simulink model "Environmentmodel"  (R2024a)
settings: Solver=VariableStepAuto  StartTime=0.0  StopTime=10.0  RelTol=1e-3
undefined symbols (not defined in the file or in its folder): F, Light, MIL, quad
libraries: shared6dof x1, aerolibwind2 x1
settings Model: Creator=akulramasubban  LastModifiedBy=akulramasubban

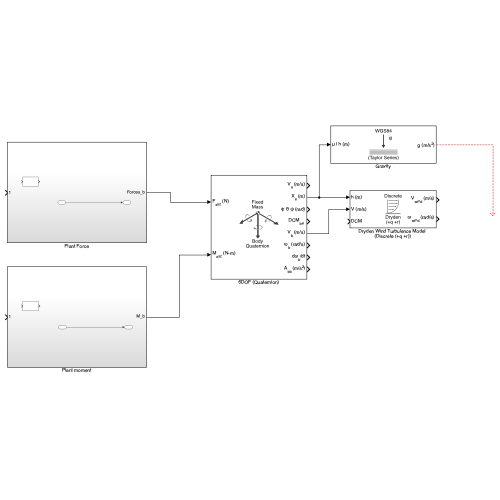
[thumbnail: Simulink's stored preview of the top-level diagram]
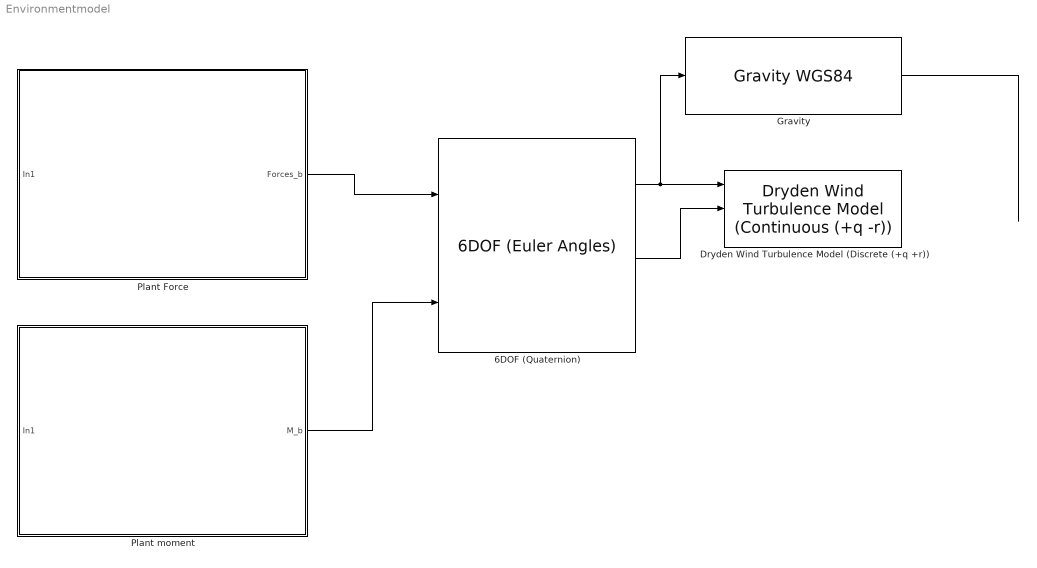
== system Environmentmodel ==
  6DOF (Quaternion) : shared6dof/6DOF (Euler Angles)  units=Metric (MKS)  mtype=Fixed  rep=Quaternion  xme_0=IC.pos  Vm_0=IC.vel  eul_0=IC.euler  pm_0=IC.omegaB  mass_0=quad  mass_e=0.5  mass_f=2.0  inertia=[quad(1,1), quad(2,2), quad(3,3)]  inertia_e=eye(3)  inertia_f=2*eye(3)  k_quat=1.0  vre_flag=on  abi_flag=off  aMode=0  xme_statename=''  Vm_statename=''  eul_statename=''  quat_statename=''  pm_statename=''  mass_statename=''
      settings: LibrarySourceBlock=aerolib6dof2/6DOF (Quaternion)
  Dryden Wind Turbulence Model (Discrete (+q +r)) : aerolibwind2/Dryden Wind Turbulence Model  (Continuous (+q -r))  units=Metric (MKS)  spec=MIL-F-8785C  model=Discrete Dryden (+q +r)  W20=15  Wdeg=0  TurbProb=10^-2 - Light  L_high=533.4  Wingspan=10  ts=0.1  Seed=[23341 23342 23343 23344]  T_on=on
      settings: LibrarySourceBlock=|
      | aerolibwind2/Dryden Wind Turbulence Model
      | (Discrete (+q +r))
  Gravity : GravityWGS84
  Plant Force : Subsystem
  Plant moment : Subsystem
  wires:
  Plant Force/1(Forces_b) -> 6DOF (Quaternion)/1
  Plant moment/1(M_b) -> 6DOF (Quaternion)/2
  Gravity/1 -> ?
  6DOF (Quaternion)/2 -> Gravity/1, Dryden Wind Turbulence Model (Discrete (+q +r))/1
  6DOF (Quaternion)/5 -> Dryden Wind Turbulence Model (Discrete (+q +r))/2

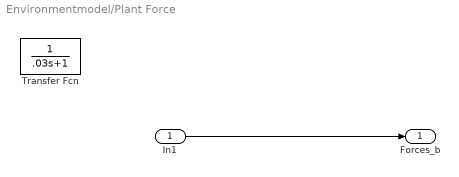
== system Environmentmodel/Plant Force ==
  In1 : Inport
  Transfer Fcn : TransferFcn  Denominator=[.03 1]
  Forces_b : Outport  Unit=N  PortDimensions=3
  wires:
  In1/1 -> Forces_b/1

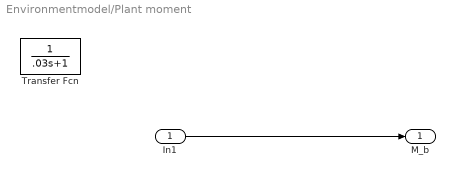
== system Environmentmodel/Plant moment ==
  In1 : Inport
  Transfer Fcn : TransferFcn  Denominator=[.03 1]
  M_b : Outport  Unit=N  PortDimensions=3
  wires:
  In1/1 -> M_b/1
